simulink model "EurlerDynJointVerify"  (Simulink 7.6)
settings: Solver=ode45  StartTime=0.0  StopTime=10  RelTol=1e-3
InitFcn:
  | eval('Config')
  | %eval('EfortConfig')
values from neighbouring files (symbols this model uses):
  a2 = 0    [Config.m]    (also in CtrPlatformCfg.m)
  a3 = 0    [Config.m]    (also in CtrPlatformCfg.m)
  a4 = 0    [Config.m]    (also in CtrPlatformCfg.m)
  a5 = 90    [Config.m]    (also in CtrPlatformCfg.m)
  a6 = 0    [Config.m]    (also in CtrPlatformCfg.m)
  Cen_EU = Cen    [DynEulerTest.m]
  DH_EU = [266     300     0       0       1016     0      174 ... (first row only)    [DynEulerTest.m]
  freq = tvel/radius    (= 1)    [Config.m]    (also in CtrPlatformCfg.m)
  Ft_EU = [0;0;0;0;0;0]    [DynEulerTest.m]
  Ie_EU = [Ie1;Ie2;Ie3;Ie4;Ie5;Ie6]    [DynEulerTest.m]
  init_Endx = gd_init(1,4)    [Config.m]    (also in CtrPlatformCfg.m)
  init_Endy = gd_init(2,4)    [Config.m]    (also in CtrPlatformCfg.m)
  init_Endz = gd_init(3,4)    [Config.m]    (also in CtrPlatformCfg.m)
  init_Rot = gd_init(1:3,1:3)    [Config.m]    (also in CtrPlatformCfg.m)
  L = [l1 l2 l3 l4 l5 l6 l7 l8 l9]    [Config.m]    (also in CtrPlatformCfg.m)
  Ma_EU = Ma    [DynEulerTest.m]
  tvel = 120    [Config.m]    (also in CtrPlatformCfg.m)
undefined symbols (not defined in the file or in its folder): a1, Cen_Min, DH_Min, Ft_Min, Ie_Min, Ma_Min
libraries: mblibv1 x41, simulink x9
(part 2 of 3)

== system EurlerDynJointVerify/Error Analysis/BodyInfoDisplay ==
  JntVel : Inport
  JntAcc : Inport  Port=2
  JntF : Inport  Port=3
  SensorBody : Inport  Port=4
  ReactionForce : Inport  Port=5
  Acc : Subsystem
  Demux : Demux  Outputs=6
  Demux{1..6,8..13} (12 alike) : Demux  Outputs=2
  Demux7 : Demux  Outputs=6
  Mux : Mux  Inputs=6
  Mux1 : Mux  Inputs=6
  Mux2 : Mux  Inputs=6
  Mux{3..8} (6 alike) : Mux  Inputs=2
  ReactionTorqueForce : Subsystem
  Vel : Subsystem
  wires:
  JntVel/1 -> Vel/1(In1)
  JntAcc/1 -> Acc/1(In1)
  SensorBody/1 -> Demux/1
  Demux/1 -> Demux1/1
  Demux/2 -> Demux2/1
  Demux/3 -> Demux3/1
  Demux/4 -> Demux4/1
  Demux/5 -> Demux5/1
  Demux/6 -> Demux6/1
  Demux1/1 -> Mux/1
  Demux2/1 -> Mux/2
  Demux3/1 -> Mux/3
  Demux4/1 -> Mux/4
  Demux5/1 -> Mux/5
  Demux6/1 -> Mux/6
  Demux1/2 -> Mux1/1
  Demux2/2 -> Mux1/2
  Demux3/2 -> Mux1/3
  Demux4/2 -> Mux1/4
  Demux5/2 -> Mux1/5
  Demux6/2 -> Mux1/6
  Mux/1 -> Vel/2(In2)
  Mux1/1 -> Acc/2(In2)
  JntF/1 -> ReactionTorqueForce/1(In1)
  Demux7/1 -> Demux8/1
  Demux7/2 -> Demux9/1
  Demux7/3 -> Demux10/1
  Demux7/4 -> Demux11/1
  Demux7/5 -> Demux12/1
  Demux7/6 -> Demux13/1
  ReactionForce/1 -> Demux7/1
  Demux8/1 -> Mux3/2
  Demux8/2 -> Mux3/1
  Demux9/1 -> Mux4/2
  Demux9/2 -> Mux4/1
  Demux10/1 -> Mux5/2
  Demux10/2 -> Mux5/1
  Demux11/1 -> Mux6/2
  Demux11/2 -> Mux6/1
  Demux12/1 -> Mux7/2
  Demux12/2 -> Mux7/1
  Demux13/1 -> Mux8/2
  Demux13/2 -> Mux8/1
  Mux3/1 -> Mux2/1
  Mux4/1 -> Mux2/2
  Mux5/1 -> Mux2/3
  Mux6/1 -> Mux2/4
  Mux7/1 -> Mux2/5
  Mux8/1 -> Mux2/6
  Mux2/1 -> ReactionTorqueForce/2(In2)

== system EurlerDynJointVerify/Error Analysis/EndTrajDisplay ==
  EnEnd : Inport
  CaEnd : Inport  Port=2
  Demux2 : Demux  Outputs=9
  Demux{20..23} (4 alike) : Demux  Outputs=3
  Demux24 : Demux  Outputs=9
  EndAcc : Scope  NumInputPorts=3
      settings: TimeRange=0.7279693486590038  YMin=-80~-80~0.03111111111111042  YMax=60~80~0.06666666666666621  SaveName=ScopeData12
  EndPos : Scope  NumInputPorts=3
      settings: TimeRange=10  YMin=1150~-100~1518.9999998  YMax=1350~200~1519.0000003  SaveName=ScopeData13
  EndVel : Scope  NumInputPorts=3
      settings: YMin=-5~-5~-5  YMax=5~5~5  SaveName=ScopeData14
  ErrAcc : Scope  NumInputPorts=3
      settings: YMin=-5~-5~-5  YMax=5~5~5  SaveName=ScopeData15
  ErrPos : Scope  NumInputPorts=3
      settings: YMin=-5~-5~-5  YMax=5~5~5  SaveName=ScopeData16
  ErrVel : Scope  NumInputPorts=3
      settings: YMin=-5~-5~-5  YMax=5~5~5  SaveName=ScopeData17
  RefAcc : Scope  NumInputPorts=3
      settings: TimeRange=10  YMin=-5~-5~-5  YMax=5~5~5  SaveName=ScopeData18
  RefPos : Scope  NumInputPorts=3
      settings: YMin=-5~-5~-5  YMax=5~5~5  SaveName=ScopeData19
  RefVel : Scope  NumInputPorts=3
      settings: TimeRange=10  YMin=0~-1~-1  YMax=60~1~1  SaveName=ScopeData20
  Sum6 : Sum  Inputs=-+|
  wires:
  EnEnd/1 -> Sum6/1, Demux24/1
  CaEnd/1 -> Sum6/2, Demux2/1
  Demux20/1 -> ErrPos/1
  Demux20/2 -> ErrPos/2
  Demux20/3 -> ErrPos/3
  Sum6/1 -> Demux22/1
  Demux22/1 -> Demux20/1
  Demux22/2 -> Demux21/1
  Demux21/1 -> ErrVel/1
  Demux21/2 -> ErrVel/2
  Demux21/3 -> ErrVel/3
  Demux2/1 -> RefPos/1
  Demux2/2 -> RefPos/2
  Demux2/3 -> RefPos/3
  Demux2/4 -> RefVel/1
  Demux2/5 -> RefVel/2
  Demux2/6 -> RefVel/3
  Demux2/7 -> RefAcc/1
  Demux2/8 -> RefAcc/2
  Demux2/9 -> RefAcc/3
  Demux23/1 -> ErrAcc/1
  Demux23/2 -> ErrAcc/2
  Demux23/3 -> ErrAcc/3
  Demux22/3 -> Demux23/1
  Demux24/1 -> EndPos/1
  Demux24/2 -> EndPos/2
  Demux24/3 -> EndPos/3
  Demux24/4 -> EndVel/1
  Demux24/5 -> EndVel/2
  Demux24/6 -> EndVel/3
  Demux24/7 -> EndAcc/1
  Demux24/8 -> EndAcc/2
  Demux24/9 -> EndAcc/3

== system EurlerDynJointVerify/Error Analysis/ForceDisplay ==
  EnForce : Inport
  CaForce : Inport  Port=2
  Demux : Demux  Outputs=6
  Demux1 : Demux  Outputs=6
  Err{1..6} (6 alike) : Scope
      Err1 settings: TimeRange=10  SaveName=ScopeData6
      Err2 settings: SaveName=ScopeData7
      Err3 settings: SaveName=ScopeData8
      Err4 settings: SaveName=ScopeData9
      Err5 settings: TimeRange=3  YMin=-2.5  YMax=1  SaveName=ScopeData10
      Err6 settings: SaveName=ScopeData11
  R1 Force : Scope  NumInputPorts=2
      settings: TimeRange=10  YMin=-2.999999999999999e-017~-1  YMax=4e-017~1
  R2 Force : Scope  NumInputPorts=2
      settings: YMin=-5~-5  YMax=5~5
  R3 Force : Scope  NumInputPorts=2
      settings: YMin=-5~-5  YMax=5~5  SaveName=ScopeData2
  R4 Force : Scope  NumInputPorts=2
      settings: YMin=-5~-5  YMax=5~5  SaveName=ScopeData3
  R5 Force : Scope  NumInputPorts=2
      settings: TimeRange=10  YMin=-4.18~4.060000000000001  YMax=-4.04~4.2  SaveName=ScopeData4
  R6 Force : Scope  NumInputPorts=2
      settings: TimeRange=10  YMin=-1.6e-006~-0.003  YMax=4e-007~0.004  SaveName=ScopeData5
  Sum{,1..5} (6 alike) : Sum  Inputs=+|-
  To Workspace : ToWorkspace  VariableName=OutEnTau  SampleTime=-1  SaveFormat=Structure
  To Workspace1 : ToWorkspace  VariableName=OutCalTau  SampleTime=-1  SaveFormat=Structure
  wires:
  Sum/1 -> Err1/1
  Sum1/1 -> Err2/1
  Sum2/1 -> Err3/1
  Sum3/1 -> Err4/1
  Sum4/1 -> Err5/1
  Sum5/1 -> Err6/1
  EnForce/1 -> Demux/1, To Workspace/1
  CaForce/1 -> Demux1/1, To Workspace1/1
  Demux/1 -> Sum/1, R1 Force/1
  Demux1/1 -> Sum/2, R1 Force/2
  Demux/2 -> R2 Force/1, Sum1/1
  Demux/3 -> R3 Force/1, Sum2/1
  Demux/4 -> Sum3/1, R4 Force/1
  Demux/5 -> R5 Force/1, Sum4/1
  Demux/6 -> R6 Force/1, Sum5/1
  Demux1/2 -> R2 Force/2, Sum1/2
  Demux1/3 -> R3 Force/2, Sum2/2
  Demux1/4 -> Sum3/2, R4 Force/2
  Demux1/5 -> R5 Force/2, Sum4/2
  Demux1/6 -> R6 Force/2, Sum5/2

== system EurlerDynJointVerify/Error Analysis/Subsystem ==
  In1 : Inport
  Demux1 : Demux  Outputs=6
  Demux{2..7} (6 alike) : Demux  Outputs=7
  Mux{,1..7} (8 alike) : Mux  Inputs=6
  Out1 : Outport
  Out2 : Outport  Port=2
  wires:
  In1/1 -> Demux1/1
  Demux1/1 -> Demux2/1
  Demux1/2 -> Demux3/1
  Demux1/3 -> Demux4/1
  Demux1/4 -> Demux5/1
  Demux1/5 -> Demux7/1
  Demux1/6 -> Demux6/1
  Demux2/1 -> Mux6/1
  Demux3/1 -> Mux6/2
  Demux4/1 -> Mux6/3
  Demux5/1 -> Mux6/4
  Demux7/1 -> Mux6/5
  Demux6/1 -> Mux6/6
  Demux2/2 -> Mux/1
  Demux2/3 -> Mux/2
  Demux2/4 -> Mux/3
  Demux2/5 -> Mux/4
  Demux2/6 -> Mux/5
  Demux2/7 -> Mux/6
  Demux3/2 -> Mux4/1
  Demux3/3 -> Mux4/2
  Demux3/4 -> Mux4/3
  Demux3/5 -> Mux4/4
  Demux3/6 -> Mux4/5
  Demux3/7 -> Mux4/6
  Demux4/2 -> Mux1/1
  Demux4/3 -> Mux1/2
  Demux4/4 -> Mux1/3
  Demux4/5 -> Mux1/4
  Demux4/6 -> Mux1/5
  Demux4/7 -> Mux1/6
  Demux5/2 -> Mux3/1
  Demux5/3 -> Mux3/2
  Demux5/4 -> Mux3/3
  Demux5/5 -> Mux3/4
  Demux5/6 -> Mux3/5
  Demux5/7 -> Mux3/6
  Demux7/2 -> Mux2/1
  Demux7/3 -> Mux2/2
  Demux7/4 -> Mux2/3
  Demux7/5 -> Mux2/4
  Demux7/6 -> Mux2/5
  Demux7/7 -> Mux2/6
  Demux6/2 -> Mux5/1
  Demux6/3 -> Mux5/2
  Demux6/4 -> Mux5/3
  Demux6/5 -> Mux5/4
  Demux6/6 -> Mux5/5
  Demux6/7 -> Mux5/6
  Mux/1 -> Mux7/1
  Mux4/1 -> Mux7/2
  Mux1/1 -> Mux7/3
  Mux3/1 -> Mux7/4
  Mux2/1 -> Mux7/5
  Mux5/1 -> Mux7/6
  Mux6/1 -> Out1/1
  Mux7/1 -> Out2/1

== system EurlerDynJointVerify/Fanuc/ BodySensor 1 ==
  Avx : Scope
      settings: TimeRange=3  YMin=-150  YMax=125  SaveName=ScopeData62
  Avy : Scope
      settings: TimeRange=3  YMin=-150  YMax=125  SaveName=ScopeData63
  Avz : Scope
      settings: TimeRange=3  YMin=-150  YMax=125  SaveName=ScopeData64
  Awx : Scope
      settings: TimeRange=3  YMin=-150  YMax=125  SaveName=ScopeData65
  Awy : Scope
      settings: TimeRange=3  YMin=-150  YMax=125  SaveName=ScopeData66
  Awz : Scope
      settings: TimeRange=3  YMin=-150  YMax=125  SaveName=ScopeData67
  "Body Sensor " : mblibv1/Sensors &  Actuators/Body Sensor  DialogController=MECH.DynMechDlgSource  SystemSampleTime=-1  UpdateFromCAD=off  PhysicalDomain=Mechanical  PortType=blob  Muxed=on  Pose=off  Angle=on  AngleUnits=deg  ArcVelocity=on  ArcVelocityUnits=deg/s  ArcAcceleration=on  ArcAccelerationUnits=deg/s^2  CoordPosition=off  CoordPositionUnits=mm  Velocity=on  VelocityUnits=mm/s  Acceleration=on  AccelerationUnits=mm/s^2  Quaternion=on  QuaternionDT=off  QuaternionDDT=off  QuaternionUnits=off  OutputVector=[1]  ActiveIO=on  Width=12  DialogClass=MechanicalSensorBlock  ReferenceFrame=Local (Body CS)
  Demux5 : Demux  Outputs=12
  Vx : Scope
      settings: TimeRange=3  YMin=-150  YMax=125  SaveName=ScopeData55
  Vy : Scope
      settings: TimeRange=3  YMin=-150  YMax=125  SaveName=ScopeData57
  Vz : Scope
      settings: TimeRange=3  YMin=-150  YMax=125  SaveName=ScopeData58
  wx : Scope
      settings: TimeRange=3  YMin=-150  YMax=125  SaveName=ScopeData59
  wy : Scope
      settings: TimeRange=3  YMin=-150  YMax=125  SaveName=ScopeData60
  wz : Scope
      settings: TimeRange=3  YMin=-150  YMax=125  SaveName=ScopeData61
  Conn1 : PMIOPort  Port=1  Side=Left
  Out : Outport
  wires:
  Demux5/12 -> Awz/1
  Demux5/11 -> Awy/1
  Demux5/10 -> Awx/1
  Demux5/9 -> Avz/1
  Demux5/8 -> Avy/1
  Demux5/7 -> Avx/1
  Demux5/6 -> wz/1
  Demux5/5 -> wy/1
  Demux5/4 -> wx/1
  Demux5/3 -> Vz/1
  Demux5/2 -> Vy/1
  Demux5/1 -> Vx/1
  "Body Sensor "/1 -> Demux5/1, Out/1
  connections:
  Conn1/RConn1 -- "Body Sensor "/LConn1

== system EurlerDynJointVerify/Fanuc/ BodySensor 2 ==
  Avx : Scope
      settings: TimeRange=3  YMin=-150  YMax=125  SaveName=ScopeData62
  Avy : Scope
      settings: TimeRange=3  YMin=-150  YMax=125  SaveName=ScopeData63
  Avz : Scope
      settings: TimeRange=3  YMin=-150  YMax=125  SaveName=ScopeData64
  Awx : Scope
      settings: TimeRange=3  YMin=-150  YMax=125  SaveName=ScopeData65
  Awy : Scope
      settings: TimeRange=3  YMin=-150  YMax=125  SaveName=ScopeData66
  Awz : Scope
      settings: TimeRange=3  YMin=-150  YMax=125  SaveName=ScopeData67
  "Body Sensor " : mblibv1/Sensors &  Actuators/Body Sensor  DialogController=MECH.DynMechDlgSource  SystemSampleTime=-1  UpdateFromCAD=off  PhysicalDomain=Mechanical  PortType=blob  Muxed=on  Pose=off  Angle=on  AngleUnits=deg  ArcVelocity=on  ArcVelocityUnits=deg/s  ArcAcceleration=on  ArcAccelerationUnits=deg/s^2  CoordPosition=off  CoordPositionUnits=mm  Velocity=on  VelocityUnits=mm/s  Acceleration=on  AccelerationUnits=mm/s^2  Quaternion=on  QuaternionDT=off  QuaternionDDT=off  QuaternionUnits=off  OutputVector=[1]  ActiveIO=on  Width=12  DialogClass=MechanicalSensorBlock  ReferenceFrame=Local (Body CS)
  Demux5 : Demux  Outputs=12
  Vx : Scope
      settings: TimeRange=3  YMin=-150  YMax=125  SaveName=ScopeData55
  Vy : Scope
      settings: TimeRange=3  YMin=-150  YMax=125  SaveName=ScopeData57
  Vz : Scope
      settings: TimeRange=3  YMin=-150  YMax=125  SaveName=ScopeData58
  wx : Scope
      settings: TimeRange=3  YMin=-150  YMax=125  SaveName=ScopeData59
  wy : Scope
      settings: TimeRange=3  YMin=-150  YMax=125  SaveName=ScopeData60
  wz : Scope
      settings: TimeRange=3  YMin=-150  YMax=125  SaveName=ScopeData61
  Conn1 : PMIOPort  Port=1  Side=Left
  Out : Outport
  wires:
  "Body Sensor "/1 -> Demux5/1, Out/1
  Demux5/1 -> Vx/1
  Demux5/2 -> Vy/1
  Demux5/3 -> Vz/1
  Demux5/4 -> wx/1
  Demux5/5 -> wy/1
  Demux5/6 -> wz/1
  Demux5/7 -> Avx/1
  Demux5/8 -> Avy/1
  Demux5/9 -> Avz/1
  Demux5/10 -> Awx/1
  Demux5/11 -> Awy/1
  Demux5/12 -> Awz/1
  connections:
  Conn1/RConn1 -- "Body Sensor "/LConn1

== system EurlerDynJointVerify/Fanuc/ BodySensor 3 ==
  Avx : Scope
      settings: TimeRange=3  YMin=-150  YMax=125  SaveName=ScopeData62
  Avy : Scope
      settings: TimeRange=3  YMin=-150  YMax=125  SaveName=ScopeData63
  Avz : Scope
      settings: TimeRange=3  YMin=-150  YMax=125  SaveName=ScopeData64
  Awx : Scope
      settings: TimeRange=3  YMin=-150  YMax=125  SaveName=ScopeData65
  Awy : Scope
      settings: TimeRange=3  YMin=-150  YMax=125  SaveName=ScopeData66
  Awz : Scope
      settings: TimeRange=3  YMin=-150  YMax=125  SaveName=ScopeData67
  "Body Sensor " : mblibv1/Sensors &  Actuators/Body Sensor  DialogController=MECH.DynMechDlgSource  SystemSampleTime=-1  UpdateFromCAD=off  PhysicalDomain=Mechanical  PortType=blob  Muxed=on  Pose=off  Angle=on  AngleUnits=deg  ArcVelocity=on  ArcVelocityUnits=deg/s  ArcAcceleration=on  ArcAccelerationUnits=deg/s^2  CoordPosition=off  CoordPositionUnits=mm  Velocity=on  VelocityUnits=mm/s  Acceleration=on  AccelerationUnits=mm/s^2  Quaternion=on  QuaternionDT=off  QuaternionDDT=off  QuaternionUnits=off  OutputVector=[1]  ActiveIO=on  Width=12  DialogClass=MechanicalSensorBlock  ReferenceFrame=Local (Body CS)
  Demux5 : Demux  Outputs=12
  Vx : Scope
      settings: TimeRange=3  YMin=-150  YMax=125  SaveName=ScopeData55
  Vy : Scope
      settings: TimeRange=3  YMin=-150  YMax=125  SaveName=ScopeData57
  Vz : Scope
      settings: TimeRange=3  YMin=-150  YMax=125  SaveName=ScopeData58
  wx : Scope
      settings: TimeRange=3  YMin=-150  YMax=125  SaveName=ScopeData59
  wy : Scope
      settings: TimeRange=3  YMin=-150  YMax=125  SaveName=ScopeData60
  wz : Scope
      settings: TimeRange=3  YMin=-150  YMax=125  SaveName=ScopeData61
  Conn1 : PMIOPort  Port=1  Side=Left
  Out : Outport
  wires:
  "Body Sensor "/1 -> Demux5/1, Out/1
  Demux5/1 -> Vx/1
  Demux5/2 -> Vy/1
  Demux5/3 -> Vz/1
  Demux5/4 -> wx/1
  Demux5/5 -> wy/1
  Demux5/6 -> wz/1
  Demux5/7 -> Avx/1
  Demux5/8 -> Avy/1
  Demux5/9 -> Avz/1
  Demux5/10 -> Awx/1
  Demux5/11 -> Awy/1
  Demux5/12 -> Awz/1
  connections:
  Conn1/RConn1 -- "Body Sensor "/LConn1

== system EurlerDynJointVerify/Fanuc/ BodySensor 4 ==
  Avx : Scope
      settings: TimeRange=3  YMin=-150  YMax=125  SaveName=ScopeData62
  Avy : Scope
      settings: TimeRange=3  YMin=-150  YMax=125  SaveName=ScopeData63
  Avz : Scope
      settings: TimeRange=3  YMin=-150  YMax=125  SaveName=ScopeData64
  Awx : Scope
      settings: TimeRange=3  YMin=-150  YMax=125  SaveName=ScopeData65
  Awy : Scope
      settings: TimeRange=3  YMin=-150  YMax=125  SaveName=ScopeData66
  Awz : Scope
      settings: TimeRange=3  YMin=-150  YMax=125  SaveName=ScopeData67
  "Body Sensor " : mblibv1/Sensors &  Actuators/Body Sensor  DialogController=MECH.DynMechDlgSource  SystemSampleTime=-1  UpdateFromCAD=off  PhysicalDomain=Mechanical  PortType=blob  Muxed=on  Pose=off  Angle=on  AngleUnits=deg  ArcVelocity=on  ArcVelocityUnits=deg/s  ArcAcceleration=on  ArcAccelerationUnits=deg/s^2  CoordPosition=off  CoordPositionUnits=mm  Velocity=on  VelocityUnits=mm/s  Acceleration=on  AccelerationUnits=mm/s^2  Quaternion=on  QuaternionDT=off  QuaternionDDT=off  QuaternionUnits=off  OutputVector=[1]  ActiveIO=on  Width=12  DialogClass=MechanicalSensorBlock  ReferenceFrame=Local (Body CS)
  Demux5 : Demux  Outputs=12
  Vx : Scope
      settings: TimeRange=3  YMin=-150  YMax=125  SaveName=ScopeData55
  Vy : Scope
      settings: TimeRange=3  YMin=-150  YMax=125  SaveName=ScopeData57
  Vz : Scope
      settings: TimeRange=3  YMin=-150  YMax=125  SaveName=ScopeData58
  wx : Scope
      settings: TimeRange=3  YMin=-150  YMax=125  SaveName=ScopeData59
  wy : Scope
      settings: TimeRange=3  YMin=-150  YMax=125  SaveName=ScopeData60
  wz : Scope
      settings: TimeRange=3  YMin=-150  YMax=125  SaveName=ScopeData61
  Conn1 : PMIOPort  Port=1  Side=Left
  Out : Outport
  wires:
  Demux5/12 -> Awz/1
  Demux5/11 -> Awy/1
  Demux5/10 -> Awx/1
  Demux5/9 -> Avz/1
  Demux5/8 -> Avy/1
  Demux5/7 -> Avx/1
  Demux5/6 -> wz/1
  Demux5/5 -> wy/1
  Demux5/4 -> wx/1
  Demux5/3 -> Vz/1
  Demux5/2 -> Vy/1
  Demux5/1 -> Vx/1
  "Body Sensor "/1 -> Demux5/1, Out/1
  connections:
  Conn1/RConn1 -- "Body Sensor "/LConn1

== system EurlerDynJointVerify/Fanuc/ BodySensor 5 ==
  Avx : Scope
      settings: TimeRange=3  YMin=-150  YMax=125  SaveName=ScopeData62
  Avy : Scope
      settings: TimeRange=3  YMin=-150  YMax=125  SaveName=ScopeData63
  Avz : Scope
      settings: TimeRange=3  YMin=-150  YMax=125  SaveName=ScopeData64
  Awx : Scope
      settings: TimeRange=3  YMin=-150  YMax=125  SaveName=ScopeData65
  Awy : Scope
      settings: TimeRange=3  YMin=-150  YMax=125  SaveName=ScopeData66
  Awz : Scope
      settings: TimeRange=3  YMin=-150  YMax=125  SaveName=ScopeData67
  "Body Sensor " : mblibv1/Sensors &  Actuators/Body Sensor  DialogController=MECH.DynMechDlgSource  SystemSampleTime=-1  UpdateFromCAD=off  PhysicalDomain=Mechanical  PortType=blob  Muxed=on  Pose=off  Angle=on  AngleUnits=deg  ArcVelocity=on  ArcVelocityUnits=deg/s  ArcAcceleration=on  ArcAccelerationUnits=deg/s^2  CoordPosition=off  CoordPositionUnits=mm  Velocity=on  VelocityUnits=mm/s  Acceleration=on  AccelerationUnits=mm/s^2  Quaternion=on  QuaternionDT=off  QuaternionDDT=off  QuaternionUnits=off  OutputVector=[1]  ActiveIO=on  Width=12  DialogClass=MechanicalSensorBlock  ReferenceFrame=Local (Body CS)
  Demux5 : Demux  Outputs=12
  Vx : Scope
      settings: TimeRange=3  YMin=-150  YMax=125  SaveName=ScopeData55
  Vy : Scope
      settings: TimeRange=3  YMin=-150  YMax=125  SaveName=ScopeData57
  Vz : Scope
      settings: TimeRange=3  YMin=-150  YMax=125  SaveName=ScopeData58
  wx : Scope
      settings: TimeRange=3  YMin=-150  YMax=125  SaveName=ScopeData59
  wy : Scope
      settings: TimeRange=3  YMin=-150  YMax=125  SaveName=ScopeData60
  wz : Scope
      settings: TimeRange=3  YMin=-150  YMax=125  SaveName=ScopeData61
  Conn1 : PMIOPort  Port=1  Side=Left
  Out : Outport
  wires:
  "Body Sensor "/1 -> Demux5/1, Out/1
  Demux5/1 -> Vx/1
  Demux5/2 -> Vy/1
  Demux5/3 -> Vz/1
  Demux5/4 -> wx/1
  Demux5/5 -> wy/1
  Demux5/6 -> wz/1
  Demux5/7 -> Avx/1
  Demux5/8 -> Avy/1
  Demux5/9 -> Avz/1
  Demux5/10 -> Awx/1
  Demux5/11 -> Awy/1
  Demux5/12 -> Awz/1
  connections:
  Conn1/RConn1 -- "Body Sensor "/LConn1

== system EurlerDynJointVerify/Fanuc/ BodySensor 6 ==
  Avx : Scope
      settings: TimeRange=3  YMin=-150  YMax=125  SaveName=ScopeData62
  Avy : Scope
      settings: TimeRange=3  YMin=-150  YMax=125  SaveName=ScopeData63
  Avz : Scope
      settings: TimeRange=3  YMin=-150  YMax=125  SaveName=ScopeData64
  Awx : Scope
      settings: TimeRange=3  YMin=-150  YMax=125  SaveName=ScopeData65
  Awy : Scope
      settings: TimeRange=3  YMin=-150  YMax=125  SaveName=ScopeData66
  Awz : Scope
      settings: TimeRange=3  YMin=-150  YMax=125  SaveName=ScopeData67
  "Body Sensor " : mblibv1/Sensors &  Actuators/Body Sensor  DialogController=MECH.DynMechDlgSource  SystemSampleTime=-1  UpdateFromCAD=off  PhysicalDomain=Mechanical  PortType=blob  Muxed=on  Pose=off  Angle=on  AngleUnits=deg  ArcVelocity=on  ArcVelocityUnits=deg/s  ArcAcceleration=on  ArcAccelerationUnits=deg/s^2  CoordPosition=off  CoordPositionUnits=mm  Velocity=on  VelocityUnits=mm/s  Acceleration=on  AccelerationUnits=mm/s^2  Quaternion=on  QuaternionDT=off  QuaternionDDT=off  QuaternionUnits=off  OutputVector=[1]  ActiveIO=on  Width=12  DialogClass=MechanicalSensorBlock  ReferenceFrame=Local (Body CS)
  Demux5 : Demux  Outputs=12
  Vx : Scope
      settings: TimeRange=3  YMin=-150  YMax=125  SaveName=ScopeData55
  Vy : Scope
      settings: TimeRange=3  YMin=-150  YMax=125  SaveName=ScopeData57
  Vz : Scope
      settings: TimeRange=3  YMin=-150  YMax=125  SaveName=ScopeData58
  wx : Scope
      settings: TimeRange=3  YMin=-150  YMax=125  SaveName=ScopeData59
  wy : Scope
      settings: TimeRange=3  YMin=-150  YMax=125  SaveName=ScopeData60
  wz : Scope
      settings: TimeRange=3  YMin=-150  YMax=125  SaveName=ScopeData61
  Conn1 : PMIOPort  Port=1  Side=Left
  Out : Outport
  wires:
  Demux5/12 -> Awz/1
  Demux5/11 -> Awy/1
  Demux5/10 -> Awx/1
  Demux5/9 -> Avz/1
  Demux5/8 -> Avy/1
  Demux5/7 -> Avx/1
  Demux5/6 -> wz/1
  Demux5/5 -> wy/1
  Demux5/4 -> wx/1
  Demux5/3 -> Vz/1
  Demux5/2 -> Vy/1
  Demux5/1 -> Vx/1
  "Body Sensor "/1 -> Demux5/1, Out/1
  connections:
  Conn1/RConn1 -- "Body Sensor "/LConn1

== system EurlerDynJointVerify/Line/EndVelocity ==
  End_Vx : Constant  Value=30
  End_Vy : Constant  Value=30
  End_Vz : Constant  Value=-30
  EndVx : Outport
  EndVy : Outport  Port=2
  EndVz : Outport  Port=3
  wires:
  End_Vx/1 -> EndVx/1
  End_Vz/1 -> EndVz/1
  End_Vy/1 -> EndVy/1

== system EurlerDynJointVerify/Line_A23/EndAngule ==
  Dot Product : DotProduct  InputSameDT=on  OutDataTypeStr=Inherit: Inherit via internal rule
  Integrator : Integrator
  R{1..2,4..6} (5 alike) : Gain  Gain=0
  R3 : Gain  Gain=0.1
  Ramp : simulink/Sources/Ramp  SystemSampleTime=-1  slope=1  start=0  X0=0
  Step : Step  After=-2  SampleTime=0
  Step1 : Step  Time=0  After=2  SampleTime=0
  Step2 : Step  SampleTime=0
  Sum : Sum  Inputs=|++
  Sum1 : Sum  Inputs=|++
  Omega1 : Outport
  Omega2 : Outport  Port=2
  Omega3 : Outport  Port=3
  Omega4 : Outport  Port=4
  Omega5 : Outport  Port=5
  Omega6 : Outport  Port=6
  wires:
  Step1/1 -> Sum1/2
  Step2/1 -> Sum/2
  Dot Product/1 -> Sum/1
  Sum1/1 -> Dot Product/1
  Step/1 -> Sum1/1
  Integrator/1 -> Dot Product/2
  Sum/1 -> R6/1, R5/1, R4/1, R3/1, R2/1, R1/1
  R1/1 -> Omega1/1
  Ramp/1 -> Integrator/1
  R2/1 -> Omega2/1
  R3/1 -> Omega3/1
  R5/1 -> Omega5/1
  R6/1 -> Omega6/1
  R4/1 -> Omega4/1

== system EurlerDynJointVerify/Line_Acc/EndAcc ==
  End_Vx : Constant  Value=0
  End_Vy : Constant  Value=0
  End_Vz : Constant  Value=0
  EndAccx : Outport
  EndAccy : Outport  Port=2
  EndAccz : Outport  Port=3
  wires:
  End_Vy/1 -> EndAccy/1
  End_Vz/1 -> EndAccz/1
  End_Vx/1 -> EndAccx/1

== system EurlerDynJointVerify/Line_JointSpace/EndAngule ==
  Dot Product : DotProduct  InputSameDT=on  OutDataTypeStr=Inherit: Inherit via internal rule
  Dot Product1 : DotProduct  InputSameDT=on  OutDataTypeStr=Inherit: Inherit via internal rule
  Dot Product2 : DotProduct  InputSameDT=on  OutDataTypeStr=Inherit: Inherit via internal rule
  Integrator : Integrator
  Integrator1 : Integrator
  Integrator2 : Integrator
  R{1..6} (6 alike) : Gain  Gain=0.05
  Ramp : simulink/Sources/Ramp  SystemSampleTime=-1  slope=1  start=0  X0=0
  Ramp1 : simulink/Sources/Ramp  SystemSampleTime=-1  slope=-1  start=0  X0=0
  Scope : Scope
      settings: SaveName=ScopeData21
  Step : Step  After=-1  SampleTime=0
  Step1 : Step  Time=0  SampleTime=0
  Step10 : Step  SampleTime=0
  Step2 : Step  Time=2  SampleTime=0
  Step3 : Step  Time=2  After=-1  SampleTime=0
  Step4 : Step  SampleTime=0
  Step5 : Step  Time=2  After=-2  SampleTime=0
  Step6 : Step  After=2  SampleTime=0
  Step7 : Step  Time=2  After=-1  SampleTime=0
  Step8 : Step  SampleTime=0
  Step9 : Step  Time=2  After=-1  SampleTime=0
  Sum : Sum  Inputs=+++
  Sum{1..2,4..6} (5 alike) : Sum  Inputs=|++
  Sum3 : Sum  Inputs=+++
  Omega1 : Outport
  Omega2 : Outport  Port=2
  Omega3 : Outport  Port=3
  Omega4 : Outport  Port=4
  Omega5 : Outport  Port=5
  Omega6 : Outport  Port=6
  wires:
  R4/1 -> Omega4/1
  R6/1 -> Omega6/1
  R5/1 -> Omega5/1
  R3/1 -> Omega3/1
  R2/1 -> Omega2/1
  Ramp/1 -> Integrator/1
  R1/1 -> Omega1/1
  Sum/1 -> R1/1, R2/1, R3/1, R4/1, R5/1, R6/1, Scope/1
  Integrator/1 -> Dot Product/2
  Step/1 -> Sum1/1
  Sum1/1 -> Dot Product/1
  Step1/1 -> Sum1/2
  Dot Product/1 -> Sum/1
  Step2/1 -> Sum/2
  Ramp1/1 -> Integrator1/1
  Integrator1/1 -> Dot Product1/2
  Step3/1 -> Sum2/1
  Sum2/1 -> Dot Product1/1
  Step4/1 -> Sum2/2
  Sum3/1 -> Sum/3
  Step5/1 -> Sum4/1
  Step6/1 -> Sum4/2
  Sum4/1 -> Integrator2/1
  Dot Product1/1 -> Sum3/2
  Step7/1 -> Sum5/1
  Step8/1 -> Sum5/2
  Sum5/1 -> Sum3/1
  Step9/1 -> Sum6/1
  Step10/1 -> Sum6/2
  Integrator2/1 -> Dot Product2/1
  Sum6/1 -> Dot Product2/2
  Dot Product2/1 -> Sum3/3

== system EurlerDynJointVerify/Still/EndVelocity ==
  Constant : Constant  Value=0
  Constant1 : Constant  Value=0
  Constant2 : Constant  Value=0
  EndVx : Outport
  EndVy : Outport  Port=2
  EndVz : Outport  Port=3
  wires:
  Constant/1 -> EndVx/1
  Constant1/1 -> EndVy/1
  Constant2/1 -> EndVz/1

== system EurlerDynJointVerify/Error Analysis/BodyInfoDisplay/Acc ==
  In1 : Inport
  In2 : Inport  Port=2
  Demux1 : Demux  Outputs=6
  Demux3 : Demux  Outputs=6
  Jnt1 : Subsystem
  Jnt2 : Subsystem
  Jnt3 : Subsystem
  Jnt4 : Subsystem
  Jnt5 : Subsystem
  Jnt6 : Subsystem
  wires:
  Demux3/6 -> Jnt6/1(In1)
  Demux3/5 -> Jnt5/1(In1)
  Demux3/4 -> Jnt4/1(In1)
  Demux3/3 -> Jnt3/1(In1)
  Demux3/2 -> Jnt2/1(In1)
  Demux3/1 -> Jnt1/1(In1)
  In1/1 -> Demux3/1
  In2/1 -> Demux1/1
  Demux1/1 -> Jnt1/2(In2)
  Demux1/2 -> Jnt2/2(In2)
  Demux1/3 -> Jnt3/2(In2)
  Demux1/4 -> Jnt4/2(In2)
  Demux1/5 -> Jnt5/2(In2)
  Demux1/6 -> Jnt6/2(In2)

== system EurlerDynJointVerify/Error Analysis/BodyInfoDisplay/ReactionTorqueForce ==
  In1 : Inport
  In2 : Inport  Port=2
  Demux1 : Demux  Outputs=6
  Demux3 : Demux  Outputs=6
  Jnt1 : Subsystem
  Jnt2 : Subsystem
  Jnt3 : Subsystem
  Jnt4 : Subsystem
  Jnt5 : Subsystem
  Jnt6 : Subsystem
  wires:
  Demux1/6 -> Jnt6/2(In2)
  Demux1/5 -> Jnt5/2(In2)
  Demux1/4 -> Jnt4/2(In2)
  Demux1/3 -> Jnt3/2(In2)
  Demux1/2 -> Jnt2/2(In2)
  Demux1/1 -> Jnt1/2(In2)
  In2/1 -> Demux1/1
  In1/1 -> Demux3/1
  Demux3/1 -> Jnt1/1(In1)
  Demux3/2 -> Jnt2/1(In1)
  Demux3/3 -> Jnt3/1(In1)
  Demux3/4 -> Jnt4/1(In1)
  Demux3/5 -> Jnt5/1(In1)
  Demux3/6 -> Jnt6/1(In1)

== system EurlerDynJointVerify/Error Analysis/BodyInfoDisplay/Vel ==
  In1 : Inport
  In2 : Inport  Port=2
  Demux1 : Demux  Outputs=6
  Demux3 : Demux  Outputs=6
  Jnt1 : Subsystem
  Jnt2 : Subsystem
  Jnt3 : Subsystem
  Jnt4 : Subsystem
  Jnt5 : Subsystem
  Jnt6 : Subsystem
  wires:
  In1/1 -> Demux3/1
  Demux3/2 -> Jnt2/1(In1)
  Demux3/3 -> Jnt3/1(In1)
  Demux3/4 -> Jnt4/1(In1)
  Demux3/5 -> Jnt5/1(In1)
  Demux3/6 -> Jnt6/1(In1)
  In2/1 -> Demux1/1
  Demux1/1 -> Jnt1/2(In2)
  Demux3/1 -> Jnt1/1(In1)
  Demux1/2 -> Jnt2/2(In2)
  Demux1/3 -> Jnt3/2(In2)
  Demux1/4 -> Jnt4/2(In2)
  Demux1/5 -> Jnt5/2(In2)
  Demux1/6 -> Jnt6/2(In2)

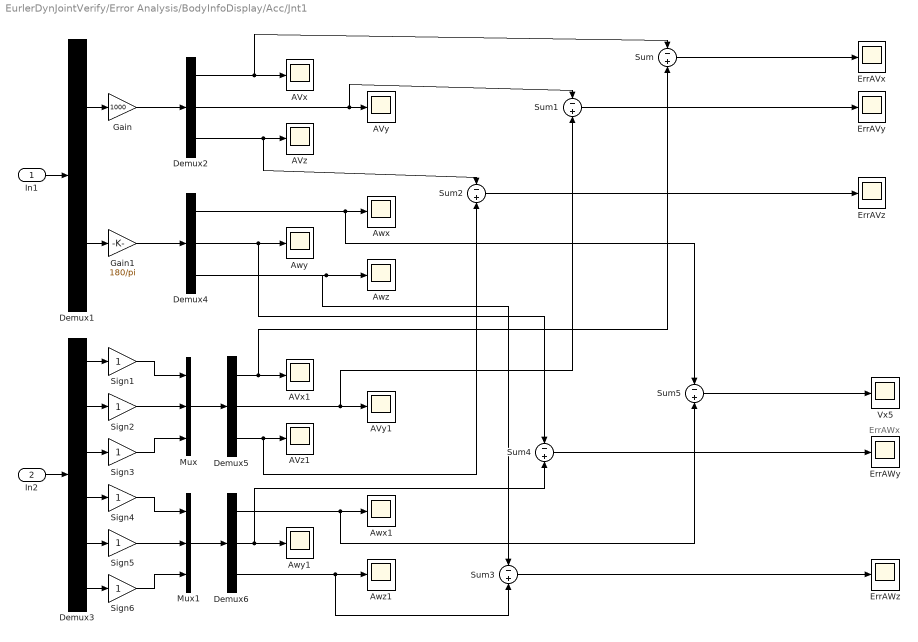
== system EurlerDynJointVerify/Error Analysis/BodyInfoDisplay/Acc/Jnt1 ==
  note: ErrAWx
  In1 : Inport
  In2 : Inport  Port=2
  AVx : Scope
      settings: TimeRange=10  YMin=-3e-017  YMax=4e-017  SaveName=ScopeData40
  AVx1 : Scope
      settings: TimeRange=10  YMin=-3e-017  YMax=4e-017  SaveName=ScopeData45
  AVy : Scope
      settings: TimeRange=10  YMin=-3e-017  YMax=4e-017  SaveName=ScopeData39
  AVy1 : Scope
      settings: TimeRange=10  YMin=-3e-017  YMax=4e-017  SaveName=ScopeData46
  AVz : Scope
      settings: TimeRange=10  YMin=-3e-017  YMax=4e-017  SaveName=ScopeData41
  AVz1 : Scope
      settings: TimeRange=10  YMin=-3e-017  YMax=4e-017  SaveName=ScopeData47
  Awx : Scope
      settings: TimeRange=3  YMin=-125  YMax=125  SaveName=ScopeData42
  Awx1 : Scope
      settings: TimeRange=3  YMin=-125  YMax=125  SaveName=ScopeData48
  Awy : Scope
      settings: TimeRange=10  YMin=-3e-017  YMax=4e-017  SaveName=ScopeData43
  Awy1 : Scope
      settings: TimeRange=10  YMin=-3e-017  YMax=4e-017  SaveName=ScopeData49
  Awz : Scope
      settings: TimeRange=10  YMin=-3e-017  YMax=4e-017  SaveName=ScopeData44
  Awz1 : Scope
      settings: TimeRange=10  YMin=-3e-017  YMax=4e-017  SaveName=ScopeData50
  Demux1 : Demux  Outputs=2
  Demux{2,4..6} (4 alike) : Demux  Outputs=3
  Demux3 : Demux  Outputs=6
  ErrAVx : Scope
      settings: TimeRange=10  YMin=-3e-017  YMax=4e-017  SaveName=ScopeData51
  ErrAVy : Scope
      settings: TimeRange=10  YMin=-3e-017  YMax=4e-017  SaveName=ScopeData52
  ErrAVz : Scope
      settings: TimeRange=10  YMin=-3e-017  YMax=4e-017  SaveName=ScopeData53
  ErrAWy : Scope
      settings: TimeRange=10  YMin=-3e-017  YMax=4e-017  SaveName=ScopeData56
  ErrAWz : Scope
      settings: TimeRange=10  YMin=-3e-017  YMax=4e-017  SaveName=ScopeData68
  Gain : Gain  Gain=1000
  Gain1 : Gain  Gain=180/pi
  Mux : Mux  Inputs=3
  Mux1 : Mux  Inputs=3
  Sign{1..6} (6 alike) : Gain
  Sum{,1..5} (6 alike) : Sum  Inputs=-|+
  Vx5 : Scope
      settings: TimeRange=10  YMin=-3e-017  YMax=4e-017  SaveName=ScopeData54
  wires:
  Sign6/1 -> Mux1/3
  Sign5/1 -> Mux1/2
  Sign4/1 -> Mux1/1
  Sign3/1 -> Mux/3
  Sign2/1 -> Mux/2
  Sign1/1 -> Mux/1
  Demux3/6 -> Sign6/1
  Demux3/5 -> Sign5/1
  Demux3/4 -> Sign4/1
  Demux3/3 -> Sign3/1
  Demux3/2 -> Sign2/1
  Demux3/1 -> Sign1/1
  Mux1/1 -> Demux6/1
  Mux/1 -> Demux5/1
  Sum/1 -> ErrAVx/1
  Sum1/1 -> ErrAVy/1
  Sum2/1 -> ErrAVz/1
  Sum3/1 -> ErrAWz/1
  Sum4/1 -> ErrAWy/1
  Sum5/1 -> Vx5/1
  In2/1 -> Demux3/1
  Demux6/3 -> Sum3/2, Awz1/1
  Demux6/2 -> Sum4/2, Awy1/1
  Demux6/1 -> Sum5/2, Awx1/1
  Demux5/3 -> Sum2/2, AVz1/1
  Demux5/2 -> Sum1/2, AVy1/1
  Demux5/1 -> Sum/2, AVx1/1
  In1/1 -> Demux1/1
  Demux4/3 -> Sum3/1, Awz/1
  Demux4/2 -> Sum4/1, Awy/1
  Demux4/1 -> Sum5/1, Awx/1
  Demux2/3 -> Sum2/1, AVz/1
  Demux2/2 -> Sum1/1, AVy/1
  Demux2/1 -> Sum/1, AVx/1
  Gain1/1 -> Demux4/1
  Gain/1 -> Demux2/1
  Demux1/2 -> Gain1/1
  Demux1/1 -> Gain/1

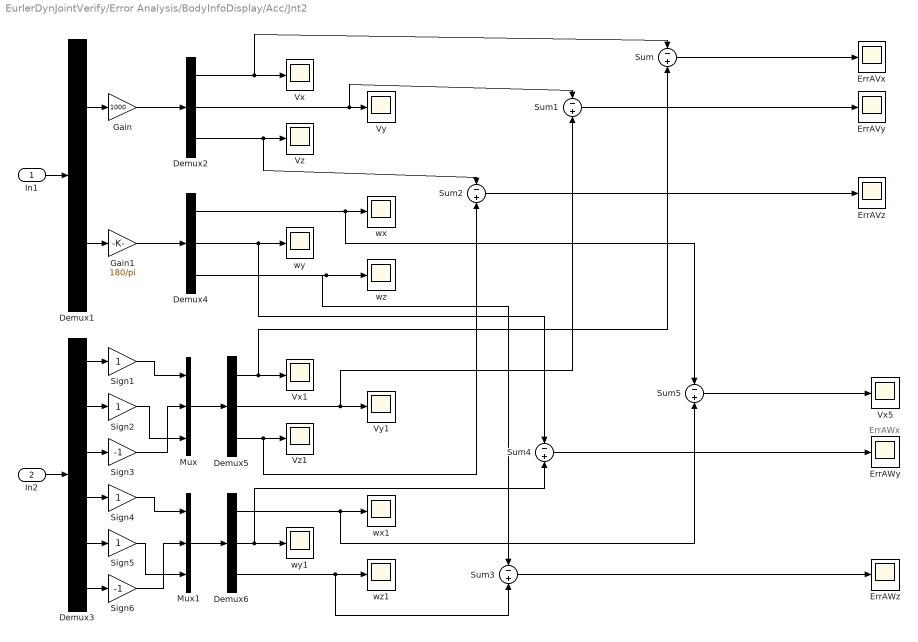
== system EurlerDynJointVerify/Error Analysis/BodyInfoDisplay/Acc/Jnt2 ==
  note: ErrAWx
  In1 : Inport
  In2 : Inport  Port=2
  Demux1 : Demux  Outputs=2
  Demux{2,4..6} (4 alike) : Demux  Outputs=3
  Demux3 : Demux  Outputs=6
  ErrAVx : Scope
      settings: TimeRange=10  YMin=-3e-017  YMax=4e-017  SaveName=ScopeData51
  ErrAVy : Scope
      settings: TimeRange=10  YMin=-3e-017  YMax=4e-017  SaveName=ScopeData52
  ErrAVz : Scope
      settings: TimeRange=10  YMin=-3e-017  YMax=4e-017  SaveName=ScopeData53
  ErrAWy : Scope
      settings: TimeRange=10  YMin=-3e-017  YMax=4e-017  SaveName=ScopeData56
  ErrAWz : Scope
      settings: TimeRange=3  YMin=-1.5e-014  YMax=1.5e-014  SaveName=ScopeData68
  Gain : Gain  Gain=1000
  Gain1 : Gain  Gain=180/pi
  Mux : Mux  Inputs=3
  Mux1 : Mux  Inputs=3
  Sign{1..2,4..5} (4 alike) : Gain
  Sign3 : Gain  Gain=-1
  Sign6 : Gain  Gain=-1
  Sum{,1..5} (6 alike) : Sum  Inputs=-|+
  Vx : Scope
      settings: TimeRange=10  YMin=-3e-017  YMax=4e-017  SaveName=ScopeData40
  Vx1 : Scope
      settings: TimeRange=10  YMin=-3e-017  YMax=4e-017  SaveName=ScopeData45
  Vx5 : Scope
      settings: TimeRange=10  YMin=-3e-017  YMax=4e-017  SaveName=ScopeData54
  Vy : Scope
      settings: TimeRange=10  YMin=-3e-017  YMax=4e-017  SaveName=ScopeData39
  Vy1 : Scope
      settings: TimeRange=10  YMin=-3e-017  YMax=4e-017  SaveName=ScopeData46
  Vz : Scope
      settings: TimeRange=10  YMin=-3e-017  YMax=4e-017  SaveName=ScopeData41
  Vz1 : Scope
      settings: TimeRange=10  YMin=-3e-017  YMax=4e-017  SaveName=ScopeData47
  wx : Scope
      settings: TimeRange=3  YMin=-125  YMax=125  SaveName=ScopeData42
  wx1 : Scope
      settings: TimeRange=3  YMin=-125  YMax=125  SaveName=ScopeData48
  wy : Scope
      settings: TimeRange=10  YMin=-3e-017  YMax=4e-017  SaveName=ScopeData43
  wy1 : Scope
      settings: TimeRange=10  YMin=-3e-017  YMax=4e-017  SaveName=ScopeData49
  wz : Scope
      settings: TimeRange=10  YMin=-3e-017  YMax=4e-017  SaveName=ScopeData44
  wz1 : Scope
      settings: TimeRange=10  YMin=-3e-017  YMax=4e-017  SaveName=ScopeData50
  wires:
  Sign5/1 -> Mux1/3
  Sign6/1 -> Mux1/2
  Sign2/1 -> Mux/3
  Sign3/1 -> Mux/2
  Demux1/1 -> Gain/1
  Demux1/2 -> Gain1/1
  Gain/1 -> Demux2/1
  Gain1/1 -> Demux4/1
  Demux2/1 -> Vx/1, Sum/1
  Demux2/2 -> Vy/1, Sum1/1
  Demux2/3 -> Vz/1, Sum2/1
  Demux4/1 -> wx/1, Sum5/1
  Demux4/2 -> wy/1, Sum4/1
  Demux4/3 -> wz/1, Sum3/1
  In1/1 -> Demux1/1
  Demux5/1 -> Vx1/1, Sum/2
  Demux5/2 -> Vy1/1, Sum1/2
  Demux5/3 -> Vz1/1, Sum2/2
  Demux6/1 -> wx1/1, Sum5/2
  Demux6/2 -> wy1/1, Sum4/2
  Demux6/3 -> wz1/1, Sum3/2
  In2/1 -> Demux3/1
  Sum5/1 -> Vx5/1
  Sum4/1 -> ErrAWy/1
  Sum3/1 -> ErrAWz/1
  Sum2/1 -> ErrAVz/1
  Sum1/1 -> ErrAVy/1
  Sum/1 -> ErrAVx/1
  Mux/1 -> Demux5/1
  Mux1/1 -> Demux6/1
  Demux3/1 -> Sign1/1
  Demux3/2 -> Sign2/1
  Demux3/3 -> Sign3/1
  Demux3/4 -> Sign4/1
  Demux3/5 -> Sign5/1
  Demux3/6 -> Sign6/1
  Sign1/1 -> Mux/1
  Sign4/1 -> Mux1/1

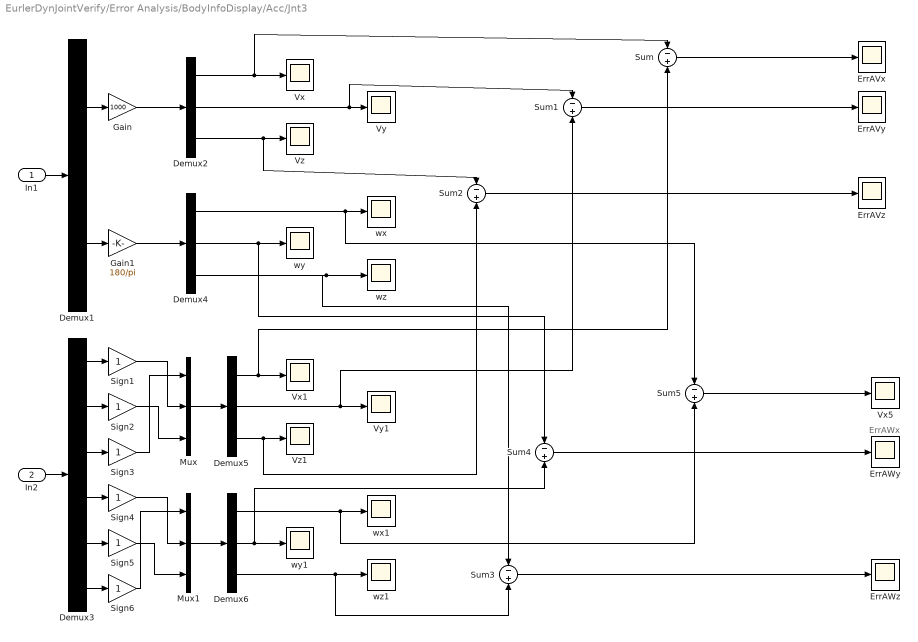
== system EurlerDynJointVerify/Error Analysis/BodyInfoDisplay/Acc/Jnt3 ==
  note: ErrAWx
  In1 : Inport
  In2 : Inport  Port=2
  Demux1 : Demux  Outputs=2
  Demux{2,4..6} (4 alike) : Demux  Outputs=3
  Demux3 : Demux  Outputs=6
  ErrAVx : Scope
      settings: TimeRange=10  YMin=-3e-017  YMax=4e-017  SaveName=ScopeData51
  ErrAVy : Scope
      settings: TimeRange=10  YMin=-3e-017  YMax=4e-017  SaveName=ScopeData52
  ErrAVz : Scope
      settings: TimeRange=10  YMin=-3e-017  YMax=4e-017  SaveName=ScopeData53
  ErrAWy : Scope
      settings: TimeRange=10  YMin=-3e-017  YMax=4e-017  SaveName=ScopeData56
  ErrAWz : Scope
      settings: TimeRange=10  YMin=-3e-017  YMax=4e-017  SaveName=ScopeData68
  Gain : Gain  Gain=1000
  Gain1 : Gain  Gain=180/pi
  Mux : Mux  Inputs=3
  Mux1 : Mux  Inputs=3
  Sign{1..6} (6 alike) : Gain
  Sum{,1..5} (6 alike) : Sum  Inputs=-|+
  Vx : Scope
      settings: TimeRange=10  YMin=-3e-017  YMax=4e-017  SaveName=ScopeData40
  Vx1 : Scope
      settings: TimeRange=10  YMin=-3e-017  YMax=4e-017  SaveName=ScopeData45
  Vx5 : Scope
      settings: TimeRange=10  YMin=-3e-017  YMax=4e-017  SaveName=ScopeData54
  Vy : Scope
      settings: TimeRange=10  YMin=-3e-017  YMax=4e-017  SaveName=ScopeData39
  Vy1 : Scope
      settings: TimeRange=10  YMin=-3e-017  YMax=4e-017  SaveName=ScopeData46
  Vz : Scope
      settings: TimeRange=10  YMin=-3e-017  YMax=4e-017  SaveName=ScopeData41
  Vz1 : Scope
      settings: TimeRange=10  YMin=-3e-017  YMax=4e-017  SaveName=ScopeData47
  wx : Scope
      settings: TimeRange=3  YMin=-125  YMax=125  SaveName=ScopeData42
  wx1 : Scope
      settings: TimeRange=3  YMin=-125  YMax=125  SaveName=ScopeData48
  wy : Scope
      settings: TimeRange=10  YMin=-3e-017  YMax=4e-017  SaveName=ScopeData43
  wy1 : Scope
      settings: TimeRange=10  YMin=-3e-017  YMax=4e-017  SaveName=ScopeData49
  wz : Scope
      settings: TimeRange=10  YMin=-3e-017  YMax=4e-017  SaveName=ScopeData44
  wz1 : Scope
      settings: TimeRange=10  YMin=-3e-017  YMax=4e-017  SaveName=ScopeData50
  wires:
  Sign6/1 -> Mux1/1
  Sign5/1 -> Mux1/3
  Sign4/1 -> Mux1/2
  Sign3/1 -> Mux/1
  Sign2/1 -> Mux/3
  Sign1/1 -> Mux/2
  Demux3/6 -> Sign6/1
  Demux3/5 -> Sign5/1
  Demux3/4 -> Sign4/1
  Demux3/3 -> Sign3/1
  Demux3/2 -> Sign2/1
  Demux3/1 -> Sign1/1
  Mux1/1 -> Demux6/1
  Mux/1 -> Demux5/1
  Sum/1 -> ErrAVx/1
  Sum1/1 -> ErrAVy/1
  Sum2/1 -> ErrAVz/1
  Sum3/1 -> ErrAWz/1
  Sum4/1 -> ErrAWy/1
  Sum5/1 -> Vx5/1
  In2/1 -> Demux3/1
  Demux6/3 -> Sum3/2, wz1/1
  Demux6/2 -> Sum4/2, wy1/1
  Demux6/1 -> Sum5/2, wx1/1
  Demux5/3 -> Sum2/2, Vz1/1
  Demux5/2 -> Sum1/2, Vy1/1
  Demux5/1 -> Sum/2, Vx1/1
  In1/1 -> Demux1/1
  Demux4/3 -> Sum3/1, wz/1
  Demux4/2 -> Sum4/1, wy/1
  Demux4/1 -> Sum5/1, wx/1
  Demux2/3 -> Sum2/1, Vz/1
  Demux2/2 -> Sum1/1, Vy/1
  Demux2/1 -> Sum/1, Vx/1
  Gain1/1 -> Demux4/1
  Gain/1 -> Demux2/1
  Demux1/2 -> Gain1/1
  Demux1/1 -> Gain/1

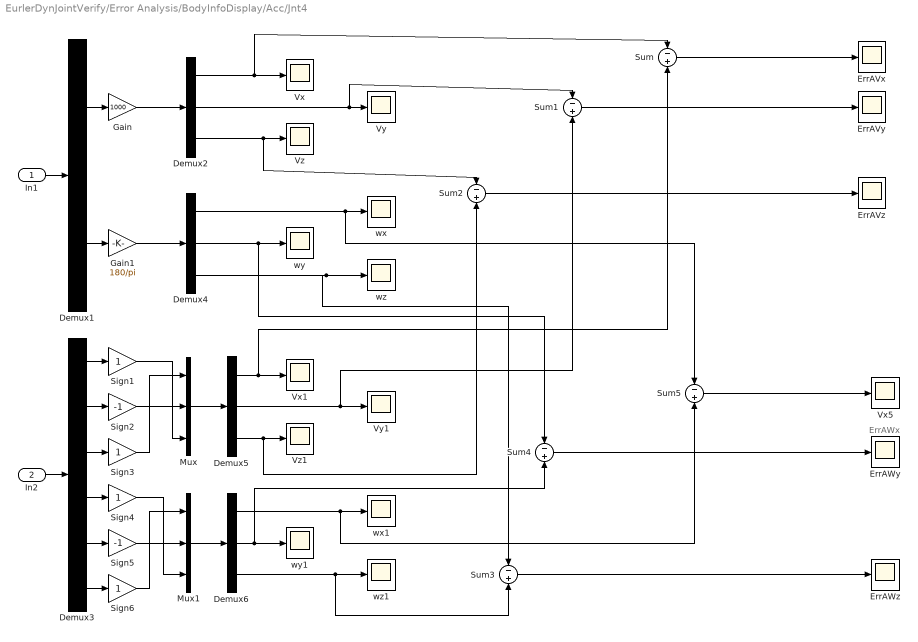
== system EurlerDynJointVerify/Error Analysis/BodyInfoDisplay/Acc/Jnt4 ==
  note: ErrAWx
  In1 : Inport
  In2 : Inport  Port=2
  Demux1 : Demux  Outputs=2
  Demux{2,4..6} (4 alike) : Demux  Outputs=3
  Demux3 : Demux  Outputs=6
  ErrAVx : Scope
      settings: TimeRange=10  YMin=-3e-017  YMax=4e-017  SaveName=ScopeData51
  ErrAVy : Scope
      settings: TimeRange=10  YMin=-3e-017  YMax=4e-017  SaveName=ScopeData52
  ErrAVz : Scope
      settings: TimeRange=10  YMin=-3e-017  YMax=4e-017  SaveName=ScopeData53
  ErrAWy : Scope
      settings: TimeRange=10  YMin=-3e-017  YMax=4e-017  SaveName=ScopeData56
  ErrAWz : Scope
      settings: TimeRange=10  YMin=-3e-017  YMax=4e-017  SaveName=ScopeData68
  Gain : Gain  Gain=1000
  Gain1 : Gain  Gain=180/pi
  Mux : Mux  Inputs=3
  Mux1 : Mux  Inputs=3
  Sign{1,3..4,6} (4 alike) : Gain
  Sign2 : Gain  Gain=-1
  Sign5 : Gain  Gain=-1
  Sum{,1..5} (6 alike) : Sum  Inputs=-|+
  Vx : Scope
      settings: TimeRange=10  YMin=-3e-017  YMax=4e-017  SaveName=ScopeData40
  Vx1 : Scope
      settings: TimeRange=10  YMin=-3e-017  YMax=4e-017  SaveName=ScopeData45
  Vx5 : Scope
      settings: TimeRange=10  YMin=-3e-017  YMax=4e-017  SaveName=ScopeData54
  Vy : Scope
      settings: TimeRange=10  YMin=-3e-017  YMax=4e-017  SaveName=ScopeData39
  Vy1 : Scope
      settings: TimeRange=10  YMin=-3e-017  YMax=4e-017  SaveName=ScopeData46
  Vz : Scope
      settings: TimeRange=10  YMin=-3e-017  YMax=4e-017  SaveName=ScopeData41
  Vz1 : Scope
      settings: TimeRange=10  YMin=-3e-017  YMax=4e-017  SaveName=ScopeData47
  wx : Scope
      settings: TimeRange=3  YMin=-125  YMax=125  SaveName=ScopeData42
  wx1 : Scope
      settings: TimeRange=3  YMin=-125  YMax=125  SaveName=ScopeData48
  wy : Scope
      settings: TimeRange=10  YMin=-3e-017  YMax=4e-017  SaveName=ScopeData43
  wy1 : Scope
      settings: TimeRange=10  YMin=-3e-017  YMax=4e-017  SaveName=ScopeData49
  wz : Scope
      settings: TimeRange=10  YMin=-3e-017  YMax=4e-017  SaveName=ScopeData44
  wz1 : Scope
      settings: TimeRange=10  YMin=-3e-017  YMax=4e-017  SaveName=ScopeData50
  wires:
  Sign6/1 -> Mux1/1
  Sign5/1 -> Mux1/2
  Sign4/1 -> Mux1/3
  Sign3/1 -> Mux/1
  Sign2/1 -> Mux/2
  Sign1/1 -> Mux/3
  Demux1/1 -> Gain/1
  Demux1/2 -> Gain1/1
  Gain/1 -> Demux2/1
  Gain1/1 -> Demux4/1
  Demux2/1 -> Vx/1, Sum/1
  Demux2/2 -> Vy/1, Sum1/1
  Demux2/3 -> Vz/1, Sum2/1
  Demux4/1 -> wx/1, Sum5/1
  Demux4/2 -> wy/1, Sum4/1
  Demux4/3 -> wz/1, Sum3/1
  In1/1 -> Demux1/1
  Demux5/1 -> Vx1/1, Sum/2
  Demux5/2 -> Vy1/1, Sum1/2
  Demux5/3 -> Vz1/1, Sum2/2
  Demux6/1 -> wx1/1, Sum5/2
  Demux6/2 -> wy1/1, Sum4/2
  Demux6/3 -> wz1/1, Sum3/2
  In2/1 -> Demux3/1
  Sum5/1 -> Vx5/1
  Sum4/1 -> ErrAWy/1
  Sum3/1 -> ErrAWz/1
  Sum2/1 -> ErrAVz/1
  Sum1/1 -> ErrAVy/1
  Sum/1 -> ErrAVx/1
  Mux/1 -> Demux5/1
  Mux1/1 -> Demux6/1
  Demux3/1 -> Sign1/1
  Demux3/2 -> Sign2/1
  Demux3/3 -> Sign3/1
  Demux3/4 -> Sign4/1
  Demux3/5 -> Sign5/1
  Demux3/6 -> Sign6/1

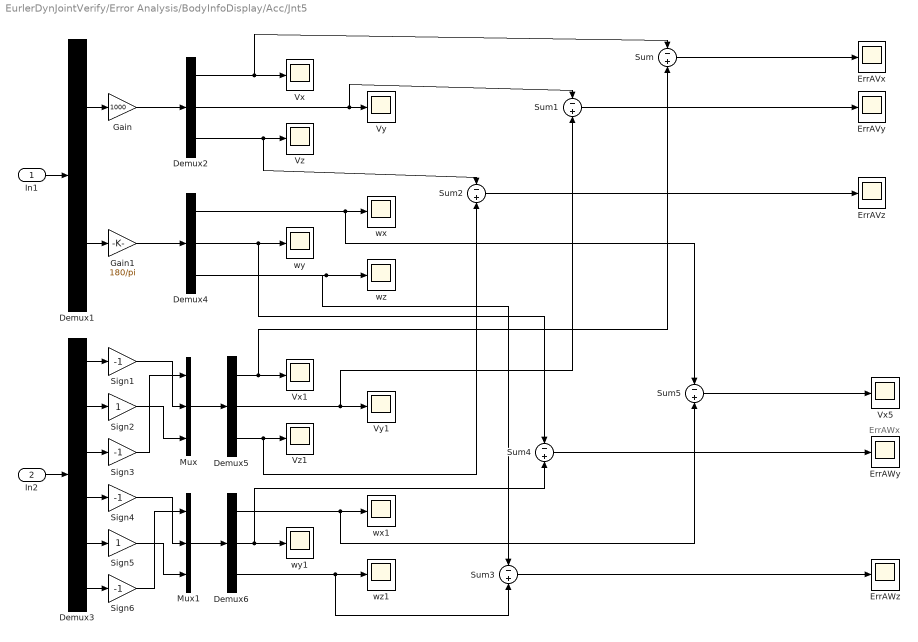
== system EurlerDynJointVerify/Error Analysis/BodyInfoDisplay/Acc/Jnt5 ==
  note: ErrAWx
  In1 : Inport
  In2 : Inport  Port=2
  Demux1 : Demux  Outputs=2
  Demux{2,4..6} (4 alike) : Demux  Outputs=3
  Demux3 : Demux  Outputs=6
  ErrAVx : Scope
      settings: TimeRange=10  YMin=-3e-017  YMax=4e-017  SaveName=ScopeData51
  ErrAVy : Scope
      settings: TimeRange=10  YMin=-3e-017  YMax=4e-017  SaveName=ScopeData52
  ErrAVz : Scope
      settings: TimeRange=10  YMin=-3e-017  YMax=4e-017  SaveName=ScopeData53
  ErrAWy : Scope
      settings: TimeRange=10  YMin=-3e-017  YMax=4e-017  SaveName=ScopeData56
  ErrAWz : Scope
      settings: TimeRange=10  YMin=-3e-017  YMax=4e-017  SaveName=ScopeData68
  Gain : Gain  Gain=1000
  Gain1 : Gain  Gain=180/pi
  Mux : Mux  Inputs=3
  Mux1 : Mux  Inputs=3
  Sign{1,3..4,6} (4 alike) : Gain  Gain=-1
  Sign2 : Gain
  Sign5 : Gain
  Sum{,1..5} (6 alike) : Sum  Inputs=-|+
  Vx : Scope
      settings: TimeRange=10  YMin=-3e-017  YMax=4e-017  SaveName=ScopeData40
  Vx1 : Scope
      settings: TimeRange=10  YMin=-3e-017  YMax=4e-017  SaveName=ScopeData45
  Vx5 : Scope
      settings: TimeRange=10  YMin=-3e-017  YMax=4e-017  SaveName=ScopeData54
  Vy : Scope
      settings: TimeRange=10  YMin=-3e-017  YMax=4e-017  SaveName=ScopeData39
  Vy1 : Scope
      settings: TimeRange=10  YMin=-3e-017  YMax=4e-017  SaveName=ScopeData46
  Vz : Scope
      settings: TimeRange=10  YMin=-3e-017  YMax=4e-017  SaveName=ScopeData41
  Vz1 : Scope
      settings: TimeRange=10  YMin=-3e-017  YMax=4e-017  SaveName=ScopeData47
  wx : Scope
      settings: TimeRange=3  YMin=-125  YMax=125  SaveName=ScopeData42
  wx1 : Scope
      settings: TimeRange=3  YMin=-125  YMax=125  SaveName=ScopeData48
  wy : Scope
      settings: TimeRange=10  YMin=-3e-017  YMax=4e-017  SaveName=ScopeData43
  wy1 : Scope
      settings: TimeRange=10  YMin=-3e-017  YMax=4e-017  SaveName=ScopeData49
  wz : Scope
      settings: TimeRange=10  YMin=-3e-017  YMax=4e-017  SaveName=ScopeData44
  wz1 : Scope
      settings: TimeRange=10  YMin=-3e-017  YMax=4e-017  SaveName=ScopeData50
  wires:
  Sign6/1 -> Mux1/1
  Sign5/1 -> Mux1/3
  Sign4/1 -> Mux1/2
  Sign3/1 -> Mux/1
  Sign2/1 -> Mux/3
  Sign1/1 -> Mux/2
  Demux3/6 -> Sign6/1
  Demux3/5 -> Sign5/1
  Demux3/4 -> Sign4/1
  Demux3/3 -> Sign3/1
  Demux3/2 -> Sign2/1
  Demux3/1 -> Sign1/1
  Mux1/1 -> Demux6/1
  Mux/1 -> Demux5/1
  Sum/1 -> ErrAVx/1
  Sum1/1 -> ErrAVy/1
  Sum2/1 -> ErrAVz/1
  Sum3/1 -> ErrAWz/1
  Sum4/1 -> ErrAWy/1
  Sum5/1 -> Vx5/1
  In2/1 -> Demux3/1
  Demux6/3 -> Sum3/2, wz1/1
  Demux6/2 -> Sum4/2, wy1/1
  Demux6/1 -> Sum5/2, wx1/1
  Demux5/3 -> Sum2/2, Vz1/1
  Demux5/2 -> Sum1/2, Vy1/1
  Demux5/1 -> Sum/2, Vx1/1
  In1/1 -> Demux1/1
  Demux4/3 -> Sum3/1, wz/1
  Demux4/2 -> Sum4/1, wy/1
  Demux4/1 -> Sum5/1, wx/1
  Demux2/3 -> Sum2/1, Vz/1
  Demux2/2 -> Sum1/1, Vy/1
  Demux2/1 -> Sum/1, Vx/1
  Gain1/1 -> Demux4/1
  Gain/1 -> Demux2/1
  Demux1/2 -> Gain1/1
  Demux1/1 -> Gain/1

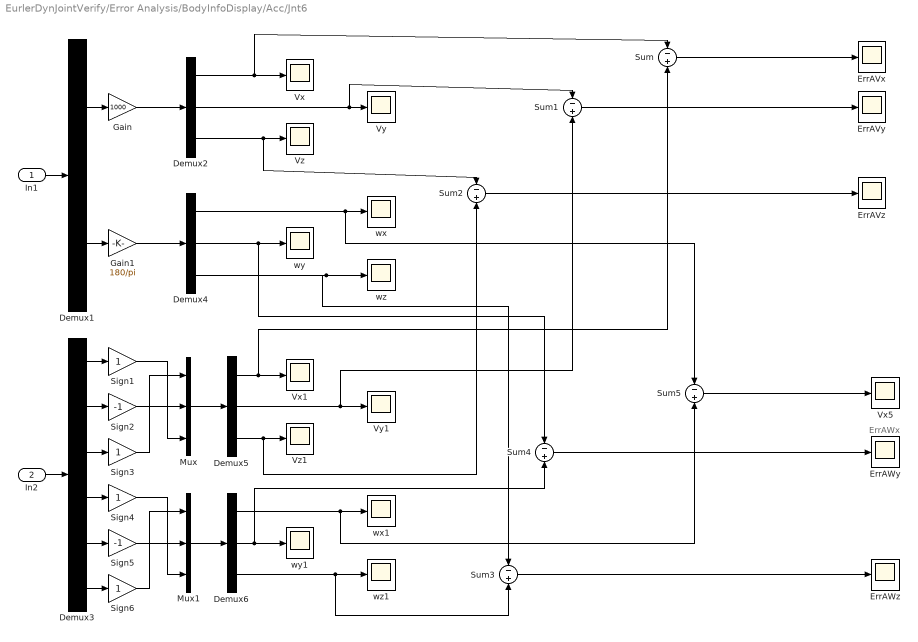
== system EurlerDynJointVerify/Error Analysis/BodyInfoDisplay/Acc/Jnt6 ==
  note: ErrAWx
  In1 : Inport
  In2 : Inport  Port=2
  Demux1 : Demux  Outputs=2
  Demux{2,4..6} (4 alike) : Demux  Outputs=3
  Demux3 : Demux  Outputs=6
  ErrAVx : Scope
      settings: TimeRange=10  YMin=-3e-017  YMax=4e-017  SaveName=ScopeData51
  ErrAVy : Scope
      settings: TimeRange=10  YMin=-3e-017  YMax=4e-017  SaveName=ScopeData52
  ErrAVz : Scope
      settings: TimeRange=10  YMin=-3e-017  YMax=4e-017  SaveName=ScopeData53
  ErrAWy : Scope
      settings: TimeRange=10  YMin=-3e-017  YMax=4e-017  SaveName=ScopeData56
  ErrAWz : Scope
      settings: TimeRange=10  YMin=-3e-017  YMax=4e-017  SaveName=ScopeData68
  Gain : Gain  Gain=1000
  Gain1 : Gain  Gain=180/pi
  Mux : Mux  Inputs=3
  Mux1 : Mux  Inputs=3
  Sign{1,3..4,6} (4 alike) : Gain
  Sign2 : Gain  Gain=-1
  Sign5 : Gain  Gain=-1
  Sum{,1..5} (6 alike) : Sum  Inputs=-|+
  Vx : Scope
      settings: TimeRange=10  YMin=-3e-017  YMax=4e-017  SaveName=ScopeData40
  Vx1 : Scope
      settings: TimeRange=10  YMin=-3e-017  YMax=4e-017  SaveName=ScopeData45
  Vx5 : Scope
      settings: TimeRange=10  YMin=-3e-017  YMax=4e-017  SaveName=ScopeData54
  Vy : Scope
      settings: TimeRange=10  YMin=-3e-017  YMax=4e-017  SaveName=ScopeData39
  Vy1 : Scope
      settings: TimeRange=10  YMin=-3e-017  YMax=4e-017  SaveName=ScopeData46
  Vz : Scope
      settings: TimeRange=10  YMin=-3e-017  YMax=4e-017  SaveName=ScopeData41
  Vz1 : Scope
      settings: TimeRange=10  YMin=-3e-017  YMax=4e-017  SaveName=ScopeData47
  wx : Scope
      settings: TimeRange=3  YMin=-125  YMax=125  SaveName=ScopeData42
  wx1 : Scope
      settings: TimeRange=3  YMin=-125  YMax=125  SaveName=ScopeData48
  wy : Scope
      settings: TimeRange=10  YMin=-3e-017  YMax=4e-017  SaveName=ScopeData43
  wy1 : Scope
      settings: TimeRange=10  YMin=-3e-017  YMax=4e-017  SaveName=ScopeData49
  wz : Scope
      settings: TimeRange=10  YMin=-3e-017  YMax=4e-017  SaveName=ScopeData44
  wz1 : Scope
      settings: TimeRange=10  YMin=-3e-017  YMax=4e-017  SaveName=ScopeData50
  wires:
  Sign6/1 -> Mux1/1
  Sign5/1 -> Mux1/2
  Sign4/1 -> Mux1/3
  Sign3/1 -> Mux/1
  Sign2/1 -> Mux/2
  Sign1/1 -> Mux/3
  Demux1/1 -> Gain/1
  Demux1/2 -> Gain1/1
  Gain/1 -> Demux2/1
  Gain1/1 -> Demux4/1
  Demux2/1 -> Vx/1, Sum/1
  Demux2/2 -> Vy/1, Sum1/1
  Demux2/3 -> Vz/1, Sum2/1
  Demux4/1 -> wx/1, Sum5/1
  Demux4/2 -> wy/1, Sum4/1
  Demux4/3 -> wz/1, Sum3/1
  In1/1 -> Demux1/1
  Demux5/1 -> Vx1/1, Sum/2
  Demux5/2 -> Vy1/1, Sum1/2
  Demux5/3 -> Vz1/1, Sum2/2
  Demux6/1 -> wx1/1, Sum5/2
  Demux6/2 -> wy1/1, Sum4/2
  Demux6/3 -> wz1/1, Sum3/2
  In2/1 -> Demux3/1
  Sum5/1 -> Vx5/1
  Sum4/1 -> ErrAWy/1
  Sum3/1 -> ErrAWz/1
  Sum2/1 -> ErrAVz/1
  Sum1/1 -> ErrAVy/1
  Sum/1 -> ErrAVx/1
  Mux/1 -> Demux5/1
  Mux1/1 -> Demux6/1
  Demux3/1 -> Sign1/1
  Demux3/2 -> Sign2/1
  Demux3/3 -> Sign3/1
  Demux3/4 -> Sign4/1
  Demux3/5 -> Sign5/1
  Demux3/6 -> Sign6/1

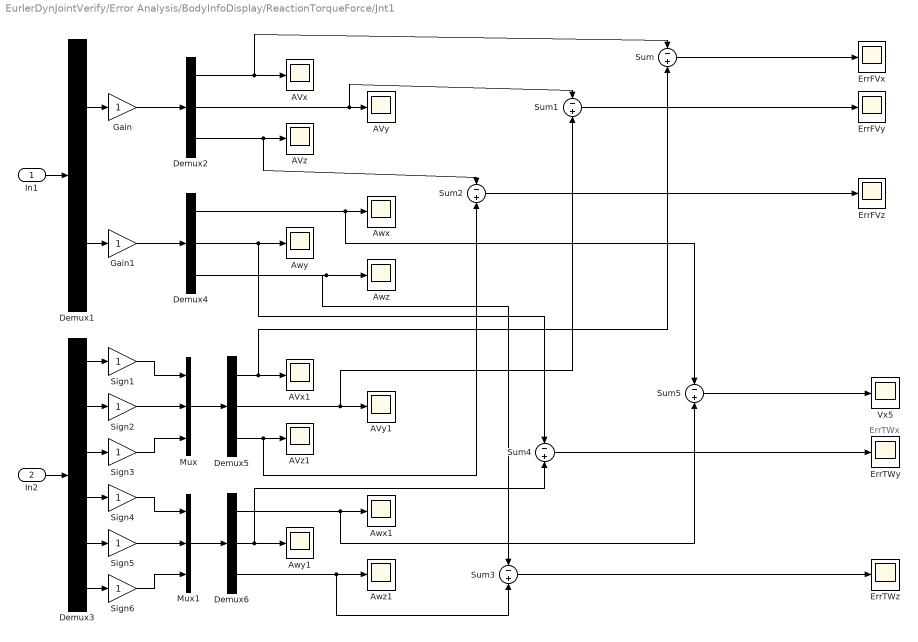
== system EurlerDynJointVerify/Error Analysis/BodyInfoDisplay/ReactionTorqueForce/Jnt1 ==
  note: ErrTWx
  In1 : Inport
  In2 : Inport  Port=2
  AVx : Scope
      settings: TimeRange=10  YMin=-3e-017  YMax=4e-017  SaveName=ScopeData40
  AVx1 : Scope
      settings: TimeRange=10  YMin=-3e-017  YMax=4e-017  SaveName=ScopeData45
  AVy : Scope
      settings: TimeRange=10  YMin=-3e-017  YMax=4e-017  SaveName=ScopeData39
  AVy1 : Scope
      settings: TimeRange=10  YMin=-3e-017  YMax=4e-017  SaveName=ScopeData46
  AVz : Scope
      settings: TimeRange=10  YMin=-3e-017  YMax=4e-017  SaveName=ScopeData41
  AVz1 : Scope
      settings: TimeRange=10  YMin=-3e-017  YMax=4e-017  SaveName=ScopeData47
  Awx : Scope
      settings: TimeRange=3  YMin=-125  YMax=125  SaveName=ScopeData42
  Awx1 : Scope
      settings: TimeRange=3  YMin=-125  YMax=125  SaveName=ScopeData48
  Awy : Scope
      settings: TimeRange=10  YMin=-3e-017  YMax=4e-017  SaveName=ScopeData43
  Awy1 : Scope
      settings: TimeRange=10  YMin=-3e-017  YMax=4e-017  SaveName=ScopeData49
  Awz : Scope
      settings: TimeRange=10  YMin=-3e-017  YMax=4e-017  SaveName=ScopeData44
  Awz1 : Scope
      settings: TimeRange=10  YMin=-3e-017  YMax=4e-017  SaveName=ScopeData50
  Demux1 : Demux  Outputs=2
  Demux{2,4..6} (4 alike) : Demux  Outputs=3
  Demux3 : Demux  Outputs=6
  ErrFVx : Scope
      settings: TimeRange=10  YMin=-3e-017  YMax=4e-017  SaveName=ScopeData51
  ErrFVy : Scope
      settings: TimeRange=10  YMin=-3e-017  YMax=4e-017  SaveName=ScopeData52
  ErrFVz : Scope
      settings: TimeRange=10  YMin=-3e-017  YMax=4e-017  SaveName=ScopeData53
  ErrTWy : Scope
      settings: TimeRange=10  YMin=-3e-017  YMax=4e-017  SaveName=ScopeData56
  ErrTWz : Scope
      settings: TimeRange=10  YMin=-3e-017  YMax=4e-017  SaveName=ScopeData68
  Gain : Gain
  Gain1 : Gain
  Mux : Mux  Inputs=3
  Mux1 : Mux  Inputs=3
  Sign{1..6} (6 alike) : Gain
  Sum{,1..5} (6 alike) : Sum  Inputs=-|+
  Vx5 : Scope
      settings: TimeRange=10  YMin=-3e-017  YMax=4e-017  SaveName=ScopeData54
  wires:
  Demux1/1 -> Gain/1
  Demux1/2 -> Gain1/1
  Gain/1 -> Demux2/1
  Gain1/1 -> Demux4/1
  Demux2/1 -> AVx/1, Sum/1
  Demux2/2 -> AVy/1, Sum1/1
  Demux2/3 -> AVz/1, Sum2/1
  Demux4/1 -> Awx/1, Sum5/1
  Demux4/2 -> Awy/1, Sum4/1
  Demux4/3 -> Awz/1, Sum3/1
  In1/1 -> Demux1/1
  Demux5/1 -> AVx1/1, Sum/2
  Demux5/2 -> AVy1/1, Sum1/2
  Demux5/3 -> AVz1/1, Sum2/2
  Demux6/1 -> Awx1/1, Sum5/2
  Demux6/2 -> Awy1/1, Sum4/2
  Demux6/3 -> Awz1/1, Sum3/2
  In2/1 -> Demux3/1
  Sum5/1 -> Vx5/1
  Sum4/1 -> ErrTWy/1
  Sum3/1 -> ErrTWz/1
  Sum2/1 -> ErrFVz/1
  Sum1/1 -> ErrFVy/1
  Sum/1 -> ErrFVx/1
  Mux/1 -> Demux5/1
  Mux1/1 -> Demux6/1
  Demux3/1 -> Sign1/1
  Demux3/2 -> Sign2/1
  Demux3/3 -> Sign3/1
  Demux3/4 -> Sign4/1
  Demux3/5 -> Sign5/1
  Demux3/6 -> Sign6/1
  Sign1/1 -> Mux/1
  Sign2/1 -> Mux/2
  Sign3/1 -> Mux/3
  Sign4/1 -> Mux1/1
  Sign5/1 -> Mux1/2
  Sign6/1 -> Mux1/3
